simulink model "TV_2017"  (R2016a)
settings: Solver=FixedStepAuto  StartTime=0.0  StopTime=inf  FixedStep=0.001  RelTol=1e-3
PreLoadFcn:
  | TV_2017_parameters
values from neighbouring files (symbols this model uses):
  battery_voltage = single(530)    [HIL_parameters.m]    (also in HIL_parameters_2018.m; TV_2017_parameters.m; TV_2017_parameters_VD.m)
  car_params = Simulink_Car_params    [HIL_parameters.m]    (also in HIL_parameters_2018.m; TV_2017_parameters.m; TV_2017_parameters_VD.m)
  i_Diff = 16    [HIL_parameters.m]    (also in HIL_parameters_2018.m; TV_2017_parameters.m)
  Kp = 1    [HIL_parameters.m]    (also in HIL_parameters_2018.m; TV_2017_parameters.m; TV_2017_parameters_VD.m)
  motor_data = struct    [HIL_parameters.m]    (also in HIL_parameters_2018.m; TV_2017_parameters.m)
  powerLimitControl = Simulink_el    [HIL_parameters.m]    (also in HIL_parameters_2018.m; TV_2017_parameters.m; TV_2017_parameters_VD.m)
  settings = Simulink_Settings    [HIL_parameters.m]    (also in HIL_parameters_2018.m; TV_2017_parameters.m; TV_2017_parameters_VD.m)
  SpdC_BCC = 0    [HIL_parameters.m]    (also in HIL_parameters_2018.m; TV_2017_parameters.m; TV_2017_parameters_VD.m)
  Speed_Neg_sat = -21    [HIL_parameters.m]    (also in HIL_parameters_2018.m; TV_2017_parameters.m; TV_2017_parameters_VD.m)
  Speed_Pos_sat = 21    [HIL_parameters.m]    (also in HIL_parameters_2018.m; TV_2017_parameters.m; TV_2017_parameters_VD.m)
  SteeringAngleFL = [-23.80 -22.65 -21.50 -20.34 -19.18 -18.03 -16.86 -15.70 -14.53 -13.35 -12.18 -10.99 -9.80 -8.61 -7.40 -6.19 -4.97 -3.75 -2.51 -1.26 0 1.27 2.56 3.85 5.17 6.50 7.84 9.21 10.59 12.00 13.42 14.88 16.36 17.87 19.41 20.99 22.61 24.26 25.97 27.73 29.54]    [CarSetupAnalysis2018.m]    (also in HIL_parameters_2018.m; TV_2017_parameters.m; TV_2017_parameters_VD.m = [-24.129 -22.950 -21.772 -20.593 -19.413 -18.232 -17.050 -15)
  SteeringAngleFR = [-29.54 -27.73 -25.97 -24.26 -22.61 -20.99 -19.41 -17.87 -16.36 -14.88 -13.42 -12.00 -10.59 -9.21 -7.84 -6.50 -5.17 -3.85 -2.56 -1.27 0 1.26 2.51 3.75 4.97 6.19 7.40 8.61 9.80 10.99 12.18 13.35 14.53 15.70 16.86 18.03 19.18 20.34 21.50 22.65 23.80]    [CarSetupAnalysis2018.m]    (also in HIL_parameters_2018.m; TV_2017_parameters.m; TV_2017_parameters_VD.m = [-29.3050 -27.5340 -25.8140 -24.1410 -22.5110 -20.9180 -19.3)
  SteeringWhAngle = [-105 -99.75 -94.5 -89.25 -84 -78.75 -73.5 -68.25 -63 -57.75 -52.5 -47.25 -42 -36.75 -31.5 -26.25 -21.0 -15.75 -10.5 -5.25 0.0 5.25 10.50 15.75 21.00 26.25 31.50 36.75 42.00 47.25 52.50 57.75  63.00 68.25 73.50 78.75 84.00 89.25 94.50 99.75 105.00]    [TV_2017_parameters_VD.m]
  Tn_n = 0    [HIL_parameters.m]    (also in HIL_parameters_2018.m; TV_2017_parameters.m; TV_2017_parameters_VD.m)
  tractionControl = Simulink_tc    [HIL_parameters.m]    (also in HIL_parameters_2018.m; IterativeTractionControlTuning.m; TV_2017_parameters.m; TV_2017_parameters_VD.m)
  yawMomentGenerator = struct    [HIL_parameters.m]    (also in HIL_parameters_2018.m = Simulink_yawRate2; TV_2017_parameters.m = Simulink_yawRate2)
  yawRateControl = Simulink_yawRate    [HIL_parameters.m]    (also in HIL_parameters_2018.m; TV_2017_parameters.m; TV_2017_parameters_VD.m)
undefined symbols (not defined in the file or in its folder): DiscIntNeverNeededParam, magnitude, speedEstimation, TC_Decr_Gas, TC_Derivative, TC_Incr_Gas, TC_On, TC_Relay_Off, TC_Relay_On
libraries: CarMaker4SL x350, simulink_extras x63, simulink x37, dspfdesign x2
(part 1 of 14)
settings Model: Creator=fh  LastModifiedBy=95fre
settings DataIOCC: LimitDataPoints=on  SaveFormat=Array  SignalLoggingSaveFormat=ModelDataLogs  SignalLoggingName=sigsOut
settings OptimizationCC: DefaultUnderspecifiedDataType=single  OptimizeBlockIOStorage=off  BufferReuse=off  GlobalBufferReuse=off  ExpressionFolding=off  ExpressionDepthLimit=2147483647  LocalBlockOutputs=off  OptimizeModelRefInitCode=on  LifeSpan=Inf  MaxStackSize=64
settings DebuggingCC: SaveWithParameterizedLinksMsg=none  UnderspecifiedInitializationDetection=Classic  SignalResolutionControl=TryResolveAllWithWarning  MultiTaskDSMMsg=warning  MultiTaskCondExecSysMsg=none  BusObjectLabelMismatch=error  ModelReferenceVersionMismatchMessage=warning  StateNameClashWarn=warning
settings HardwareCC: ProdBitPerPointer=32  ProdLargestAtomicInteger=Long  ProdLargestAtomicFloat=Double  ProdWordSize=32  ProdHWDeviceType=ARM Compatible->ARM Cortex  TargetLargestAtomicInteger=Long  TargetLargestAtomicFloat=Double  TargetEndianess=LittleEndian  TargetHWDeviceType=ARM Compatible->ARM Cortex
settings ModelReferenceCC: PropagateSignalLabelsOutOfModel=off
settings RTWCC: SystemTargetFile=ert.tlc  GenCodeOnly=on  TemplateMakefile=ert_default_tmf  GenerateReport=on  Toolchain=GNU Tools for ARM Embedded Processors  BuildConfiguration=Debug  IncludeHyperlinkInReport=on  LaunchReport=on
settings CodeAppCC: ForceParamTrailComments=on  IgnoreCustomStorageClasses=off  SimulinkDataObjDesc=on  SFDataObjDesc=on  MATLABFcnDesc=on  InsertBlockDesc=on  MATLABSourceComments=on  EnableCustomComments=on  ReqsInCode=on
settings ERTTargetCC: GenerateSampleERTMain=on  IncludeMdlTerminateFcn=off  MatFileLogging=on  SupportNonFinite=off  SupportComplex=off  SupportVariableSizeSignals=on  ERTCustomFileTemplate=example_file_process.tlc  SuppressUnreachableDefaultCases=off
settings ConfigComp: CovHTMLOptions=-sRT=1 -sVT=0 -aTS=1 -bRG=1 -bTC=1 -hTR=0 -nFC=0 -nFD=1 -scm=1 -bcm=1 -xEv=0 -xEM=0  CovModelRefEnable=Off  PSAutoStubLUT=off

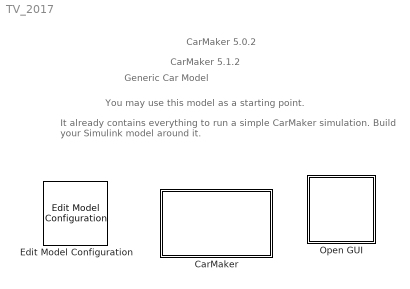
== system TV_2017 ==
  note: Generic Car Model
  note: You may use this model as a starting point.
  note: It already contains everything to run a simple CarMaker simulation.
      | Build your Simulink model around it.
  note: CarMaker 5.0.2
  note: CarMaker 5.1.2
  CarMaker : Subsystem  TreatAsAtomicUnit=on
      mask Display: image(imread('CarMakerSys.png'));
  Edit Model Configuration : CarMaker4SL/Edit Model Configuration
  Open GUI : Subsystem  LoadFcn=if ~length(which('cmcmd')), cmenv; end
      settings: OpenFcn=cmblockmagic('gui_fix_display'); CM_Simulink
      mask Display: image('CarMakerGUI.png');

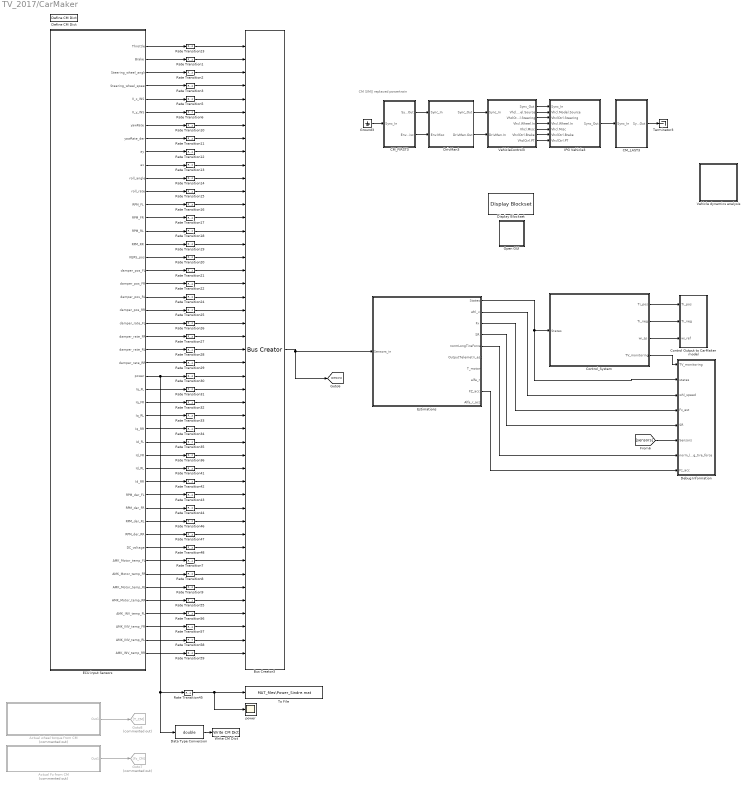
== system TV_2017/CarMaker ==
  note: CM SIM|| replaced powertrain
  Actual Fz from CM : Subsystem  Commented=on
  Actual wheel torque from CM : Subsystem  Commented=on
  Bus Creator3 : BusCreator  Inputs=47  OutDataTypeStr=Bus: SensorInputs  NonVirtualBus=on
      settings: InheritFromInputs=off
  CM_FIRST3 : Subsystem
  CM_LAST3 : Subsystem
  "Control Output to CarMaker model " : Subsystem
  "Control_System " : Subsystem  TreatAsAtomicUnit=on
  Data Type Conversion : DataTypeConversion  OutDataTypeStr=double
  "Debug Information " : Subsystem
  Define CM Dict : CarMaker4SL/Define CM Dict  xname=Power  xmono=off  xtype=Double  xdvaplace=None  xnstates=0  xfirststate=0  xinitial=0
  Display Blockset : CarMaker4SL/Display Blockset
  DrivMan3 : Subsystem
  "ECU input Sensors " : Subsystem  SystemSampleTime=settings.control_system_sample_time
  Estimations : Subsystem  TreatAsAtomicUnit=on
  Goto7 : Goto  Commented=on  GotoTag=Fz_CM
  Goto8 : Goto  Commented=on  GotoTag=T_CM
  Ground3 : Ground
  IPG Vehicle3 : Subsystem  TreatAsAtomicUnit=on
  Open GUI : Subsystem  LoadFcn=if ~length(which('cmcmd')), cmenv; end
      settings: OpenFcn=cmblockmagic('gui_fix_display'); CM_Simulink
      mask Display: image('CarMakerGUI.png');
  Rate Transition{1..3,5..36,41..48,55..59} (48 alike) : RateTransition  OutPortSampleTime=matlab_params.sensor_sampling_time
  Terminator3 : Terminator
  To File : ToFile  Filename=MAT_files\Power_Sindre.mat  MatrixName=Power  SaveFormat=Timeseries
  Vehicle dynamics analysis : Subsystem
  VehicleControl3 : Subsystem
  Write CM Dict : CarMaker4SL/Write CM Dict  xname=Power  xsync=off
  power : Scope
  wires:
  "Control_System "/1("Ti_pos ") -> "Control Output to CarMaker model "/1("Ti_pos ")
  "Control_System "/2(Ti_neg) -> "Control Output to CarMaker model "/2(Ti_neg)
  "Control_System "/3(wi_sp) -> "Control Output to CarMaker model "/3(wi_ref)
  Estimations/1(States) -> "Control_System "/1("States "), "Debug Information "/2(states)
  Estimations/2(whl_v) -> "Debug Information "/3(whl_speed)
  Estimations/3(Fx) -> "Debug Information "/4(Fx_est)
  Estimations/4(SR) -> "Debug Information "/5("SR ")
  Rate Transition45/1 -> power/1, To File/1
  "ECU input Sensors "/37(RPM_der_RL) -> Rate Transition46/1
  "ECU input Sensors "/38(RPM_der_RR) -> Rate Transition47/1
  "ECU input Sensors "/36(RPM_der_FR) -> Rate Transition44/1
  "ECU input Sensors "/35(RPM_der_FL) -> Rate Transition43/1
  "ECU input Sensors "/34(Id_RR) -> Rate Transition42/1
  "ECU input Sensors "/4(Steering_wheel_speed) -> Rate Transition3/1
  "ECU input Sensors "/1("Throttle ") -> Rate Transition23/1
  "ECU input Sensors "/2("Brake ") -> Rate Transition1/1
  "ECU input Sensors "/3("Steering_wheel_angle ") -> Rate Transition2/1
  "ECU input Sensors "/5(V_x_INS) -> Rate Transition5/1
  "ECU input Sensors "/6(V_y_INS) -> Rate Transition6/1
  "ECU input Sensors "/7(yawRate) -> Rate Transition10/1
  "ECU input Sensors "/9(ay) -> Rate Transition12/1
  "ECU input Sensors "/10("ax ") -> Rate Transition13/1
  "ECU input Sensors "/11(roll_angle) -> Rate Transition14/1
  "ECU input Sensors "/12(roll_rate) -> Rate Transition15/1
  "ECU input Sensors "/13(RPM_FL) -> Rate Transition16/1
  "ECU input Sensors "/14(RPM_FR) -> Rate Transition17/1
  "ECU input Sensors "/15(RPM_RL) -> Rate Transition18/1
  "ECU input Sensors "/16(RPM_RR) -> Rate Transition19/1
  "ECU input Sensors "/17(KERS_pos) -> Rate Transition20/1
  "ECU input Sensors "/18(damper_pos_FL) -> Rate Transition21/1
  "ECU input Sensors "/19(damper_pos_FR) -> Rate Transition22/1
  "ECU input Sensors "/20(damper_pos_RL) -> Rate Transition24/1
  "ECU input Sensors "/21(damper_pos_RR) -> Rate Transition25/1
  "ECU input Sensors "/22(damper_rate_FL) -> Rate Transition26/1
  "ECU input Sensors "/23(damper_rate_FR) -> Rate Transition27/1
  "ECU input Sensors "/24(damper_rate_RL) -> Rate Transition28/1
  "ECU input Sensors "/25(damper_rate_RR) -> Rate Transition29/1
  "ECU input Sensors "/27(Iq_FL) -> Rate Transition31/1
  "ECU input Sensors "/28(Iq_FR) -> Rate Transition32/1
  "ECU input Sensors "/29(Iq_RL) -> Rate Transition33/1
  "ECU input Sensors "/30(Iq_RR) -> Rate Transition34/1
  "ECU input Sensors "/31(Id_FL) -> Rate Transition35/1
  "ECU input Sensors "/32(Id_FR) -> Rate Transition36/1
  "ECU input Sensors "/33(Id_RL) -> Rate Transition41/1
  "ECU input Sensors "/8(yawRate_der) -> Rate Transition11/1
  "ECU input Sensors "/39(DC_voltage) -> Rate Transition48/1
  Rate Transition23/1 -> Bus Creator3/1
  Estimations/5(normLongTireForce) -> "Debug Information "/7(norm_long_tire_force)
  Rate Transition17/1 -> Bus Creator3/14
  Rate Transition12/1 -> Bus Creator3/9
  Rate Transition30/1 -> Bus Creator3/26
  Rate Transition14/1 -> Bus Creator3/11
  Rate Transition16/1 -> Bus Creator3/13
  Rate Transition25/1 -> Bus Creator3/21
  Rate Transition3/1 -> Bus Creator3/4
  Rate Transition2/1 -> Bus Creator3/3
  Rate Transition22/1 -> Bus Creator3/19
  Rate Transition11/1 -> Bus Creator3/8
  Rate Transition18/1 -> Bus Creator3/15
  Rate Transition20/1 -> Bus Creator3/17
  Rate Transition1/1 -> Bus Creator3/2
  Rate Transition24/1 -> Bus Creator3/20
  Rate Transition31/1 -> Bus Creator3/27
  Rate Transition26/1 -> Bus Creator3/22
  Rate Transition29/1 -> Bus Creator3/25
  Rate Transition15/1 -> Bus Creator3/12
  Rate Transition13/1 -> Bus Creator3/10
  Rate Transition28/1 -> Bus Creator3/24
  Rate Transition19/1 -> Bus Creator3/16
  Rate Transition21/1 -> Bus Creator3/18
  Rate Transition27/1 -> Bus Creator3/23
  Rate Transition6/1 -> Bus Creator3/6
  Rate Transition42/1 -> Bus Creator3/34
  Rate Transition47/1 -> Bus Creator3/38
  Rate Transition48/1 -> Bus Creator3/39
  Rate Transition41/1 -> Bus Creator3/33
  Rate Transition43/1 -> Bus Creator3/35
  Rate Transition35/1 -> Bus Creator3/31
  Rate Transition34/1 -> Bus Creator3/30
  Rate Transition46/1 -> Bus Creator3/37
  Rate Transition44/1 -> Bus Creator3/36
  Rate Transition33/1 -> Bus Creator3/29
  Rate Transition32/1 -> Bus Creator3/28
  Rate Transition36/1 -> Bus Creator3/32
  Rate Transition10/1 -> Bus Creator3/7
  Bus Creator3/1 -> [sensors], Estimations/1(Sensors_in)
  "ECU input Sensors "/26(power) -> Data Type Conversion/1, Rate Transition45/1, Rate Transition30/1
  Data Type Conversion/1 -> Write CM Dict/1
  [sensors] -> "Debug Information "/6(Sensors)
  "ECU input Sensors "/44(AMK_INV_temp_FL) -> Rate Transition56/1
  "ECU input Sensors "/40(AMK_Motor_temp_FL) -> Rate Transition7/1
  "ECU input Sensors "/41(AMK_Motor_temp_FR) -> Rate Transition8/1
  "ECU input Sensors "/42(AMK_Motor_temp_RL) -> Rate Transition9/1
  "ECU input Sensors "/43(AMK_Motor_temp_RR) -> Rate Transition55/1
  "ECU input Sensors "/45(AMK_INV_temp_FR) -> Rate Transition57/1
  "ECU input Sensors "/46(AMK_INV_temp_RL) -> Rate Transition58/1
  "ECU input Sensors "/47(AMK_INV_temp_RR) -> Rate Transition59/1
  Rate Transition7/1 -> Bus Creator3/40
  Rate Transition8/1 -> Bus Creator3/41
  Rate Transition9/1 -> Bus Creator3/42
  Rate Transition55/1 -> Bus Creator3/43
  Rate Transition56/1 -> Bus Creator3/44
  Rate Transition57/1 -> Bus Creator3/45
  Rate Transition58/1 -> Bus Creator3/46
  Rate Transition59/1 -> Bus Creator3/47
  Actual wheel torque from CM/1(Out1) -> Goto8/1
  Actual Fz from CM/1(Out1) -> Goto7/1
  "Control_System "/4(TV_monitoring) -> "Debug Information "/1(TV_monitoring)
  VehicleControl3/7(VhclCtrl.PT) -> IPG Vehicle3/7(VhclCtrl.PT)
  VehicleControl3/6(VhclCtrl.Brake) -> IPG Vehicle3/6(VhclCtrl.Brake)
  CM_FIRST3/1(Sync_Out) -> DrivMan3/1(Sync_In)
  CM_FIRST3/2(Env.Misc) -> DrivMan3/2(Env.Misc)
  VehicleControl3/3(VhclCtrl.Steering) -> IPG Vehicle3/3(VhclCtrl.Steering)
  DrivMan3/2(DrivMan.Out) -> VehicleControl3/2(DrivMan.In)
  VehicleControl3/2(Vhcl.Model.Source) -> IPG Vehicle3/2(Vhcl.Model.Source)
  VehicleControl3/5(Vhcl.Misc) -> IPG Vehicle3/5(Vhcl.Misc)
  VehicleControl3/1(Sync_Out) -> IPG Vehicle3/1(Sync_In)
  VehicleControl3/4(Vhcl.Wheel.In) -> IPG Vehicle3/4(Vhcl.Wheel.In)
  DrivMan3/1(Sync_Out) -> VehicleControl3/1(Sync_In)
  Ground3/1 -> CM_FIRST3/1(Sync_In)
  IPG Vehicle3/1(Sync_Out) -> CM_LAST3/1(Sync_In)
  CM_LAST3/1(Sync_Out) -> Terminator3/1
  Estimations/9(FZ_acc) -> "Debug Information "/8(Fz_acc)
  Rate Transition5/1 -> Bus Creator3/5

== system TV_2017/Open GUI ==
  S-Function : S-Function  FunctionName=cm_gui  SFunctionDeploymentMode=off  EnableBusSupport=off

== system TV_2017/CarMaker/Actual Fz from CM ==
  Bus Creator1 : BusCreator  Inputs=4
  Bus Creator4 : BusCreator  Inputs=4  OutDataTypeStr=Bus: normalForces  NonVirtualBus=on
      settings: InheritFromInputs=off
  Data Type Conversion{4..11} (8 alike) : DataTypeConversion  OutDataTypeStr=single
  Divide{,1..3} (4 alike) : Product  Inputs=*/
  Friction : Scope
  Rate Transition4 : RateTransition  OutPortSampleTime=matlab_params.sensor_sampling_time
  Read CM Dict10 : CarMaker4SL/Read CM Dict  xname=Vhcl.RL.Fx  xsync=off
  Read CM Dict11 : CarMaker4SL/Read CM Dict  xname=Vhcl.RR.Fx  xsync=off
  Read CM Dict3 : CarMaker4SL/Read CM Dict  xname=Vhcl.FR.Fz  xsync=off
  Read CM Dict4 : CarMaker4SL/Read CM Dict  xname=Vhcl.FL.Fz  xsync=off
  Read CM Dict5 : CarMaker4SL/Read CM Dict  xname=Vhcl.RR.Fz  xsync=off
  Read CM Dict6 : CarMaker4SL/Read CM Dict  xname=Vhcl.RL.Fz  xsync=off
  Read CM Dict8 : CarMaker4SL/Read CM Dict  xname=Vhcl.FL.Fx  xsync=off
  Read CM Dict9 : CarMaker4SL/Read CM Dict  xname=Vhcl.FR.Fx  xsync=off
  Out1 : Outport
  wires:
  Rate Transition4/1 -> Out1/1
  Read CM Dict4/1 -> Data Type Conversion4/1
  Read CM Dict5/1 -> Data Type Conversion7/1
  Read CM Dict3/1 -> Data Type Conversion5/1
  Read CM Dict6/1 -> Data Type Conversion6/1
  Data Type Conversion7/1 -> Bus Creator4/4, Divide3/2
  Data Type Conversion5/1 -> Bus Creator4/2, Divide1/2
  Data Type Conversion6/1 -> Bus Creator4/3, Divide2/2
  Divide/1 -> Bus Creator1/1  "FL"
  Read CM Dict10/1 -> Data Type Conversion10/1
  Data Type Conversion11/1 -> Divide3/1
  Data Type Conversion9/1 -> Divide1/1
  Data Type Conversion8/1 -> Divide/1
  Read CM Dict9/1 -> Data Type Conversion9/1
  Read CM Dict11/1 -> Data Type Conversion11/1
  Divide3/1 -> Bus Creator1/4  "RR"
  Bus Creator1/1 -> Friction/1
  Data Type Conversion4/1 -> Bus Creator4/1, Divide/2
  Read CM Dict8/1 -> Data Type Conversion8/1
  Divide2/1 -> Bus Creator1/3  "RL"
  Bus Creator4/1 -> Rate Transition4/1
  Data Type Conversion10/1 -> Divide2/1
  Divide1/1 -> Bus Creator1/2  "FR"

== system TV_2017/CarMaker/Actual wheel torque from CM ==
  Bus Creator2 : BusCreator  Inputs=4  OutDataTypeStr=Bus: T_meas
      settings: InheritFromInputs=off
  Data Type Conversion{1..3,12..15} (7 alike) : DataTypeConversion  OutDataTypeStr=single
  Rate Transition{37..40} (4 alike) : RateTransition  OutPortSampleTime=matlab_params.sensor_sampling_time
  Read CM Dict1 : CarMaker4SL/Read CM Dict  xname=Car.DampFL.Frc_tot  xsync=off
  Read CM Dict12 : CarMaker4SL/Read CM Dict  xname=PT.WFL.Trq_Drive  xsync=off
  Read CM Dict2 : CarMaker4SL/Read CM Dict  xname=Car.SpringFL.Frc_tot  xsync=off
  Read CM Dict45 : CarMaker4SL/Read CM Dict  xname=PT.WFR.Trq_Drive  xsync=off
  Read CM Dict46 : CarMaker4SL/Read CM Dict  xname=PT.WRL.Trq_Drive  xsync=off
  Read CM Dict47 : CarMaker4SL/Read CM Dict  xname=PT.WRR.Trq_Drive  xsync=off
  Read CM Dict7 : CarMaker4SL/Read CM Dict  xname=Car.StabiFL.Frc_tot  xsync=off
  "damp force fl " : Scope
  spring force fl : Scope
  spring force fl1 : Scope
  Out1 : Outport
  wires:
  Bus Creator2/1 -> Out1/1
  Rate Transition38/1 -> Bus Creator2/2
  Data Type Conversion1/1 -> "damp force fl "/1
  Data Type Conversion2/1 -> spring force fl/1
  Data Type Conversion3/1 -> spring force fl1/1
  Read CM Dict2/1 -> Data Type Conversion2/1
  Read CM Dict7/1 -> Data Type Conversion3/1
  Read CM Dict1/1 -> Data Type Conversion1/1
  Data Type Conversion12/1 -> Rate Transition37/1  "FL"
  Data Type Conversion14/1 -> Rate Transition39/1  "RL"
  Read CM Dict46/1 -> Data Type Conversion14/1
  Rate Transition39/1 -> Bus Creator2/3
  Data Type Conversion15/1 -> Rate Transition40/1  "RR"
  Read CM Dict12/1 -> Data Type Conversion12/1
  Read CM Dict47/1 -> Data Type Conversion15/1
  Rate Transition37/1 -> Bus Creator2/1
  Rate Transition40/1 -> Bus Creator2/4
  Read CM Dict45/1 -> Data Type Conversion13/1
  Data Type Conversion13/1 -> Rate Transition38/1  "FR"

== system TV_2017/CarMaker/CM_FIRST3 ==
  Sync_In : Inport
  BusCreator1 : BusCreator  Inputs=8
  BusCreator2 : BusCreator  Inputs=6
  Demux1 : Demux  Outputs=14
  Environment : S-Function  FunctionName=CM_Sfun  Parameters='Environment'  SFunctionDeploymentMode=off  EnableBusSupport=off
  IoIn : S-Function  FunctionName=CM_Sfun  Parameters='IoIn'  SFunctionDeploymentMode=off  EnableBusSupport=off
  Terminator : Terminator
  Sync_Out : Outport
  Env.Misc : Outport  Port=2
  wires:
  BusCreator2/1 -> Terminator/1  "IF Environment (in)"
  BusCreator1/1 -> Env.Misc/1
  Demux1/14 -> BusCreator2/6  "Env sRoad"
  Demux1/13 -> BusCreator2/5  "Env PoI_GCS Elev"
  Demux1/12 -> BusCreator2/4  "Env PoI_GCS Lat"
  Demux1/11 -> BusCreator2/3  "Env PoI_GCS Long"
  Demux1/10 -> BusCreator2/2  "Env Time"
  Demux1/9 -> BusCreator2/1  "Env yDay"
  Demux1/8 -> BusCreator1/8  "Env WindVel_tot z"
  Demux1/7 -> BusCreator1/7  "Env WindVel_tot y"
  Demux1/6 -> BusCreator1/6  "Env WindVel_tot x"
  Demux1/5 -> BusCreator1/5  "Env SolarRadiation"
  Demux1/4 -> BusCreator1/4  "Env AirHumidity"
  Demux1/3 -> BusCreator1/3  "Env AirPressure"
  Demux1/2 -> BusCreator1/2  "Env AirDensity"
  Demux1/1 -> BusCreator1/1  "Env Temperature"
  Environment/2 -> Demux1/1
  Environment/1 -> Sync_Out/1
  IoIn/1 -> Environment/1
  Sync_In/1 -> IoIn/1

== system TV_2017/CarMaker/CM_LAST3 ==
  Sync_In : Inport
  CM_User : S-Function  FunctionName=CM_Sfun  Parameters='CM_User'  SFunctionDeploymentMode=off  EnableBusSupport=off
  IoOut : S-Function  FunctionName=CM_Sfun  Parameters='IoOut'  SFunctionDeploymentMode=off  EnableBusSupport=off
  Sync_Out : Outport
  wires:
  IoOut/1 -> Sync_Out/1
  CM_User/1 -> IoOut/1
  Sync_In/1 -> CM_User/1

== system TV_2017/CarMaker/Control Output to CarMaker model  ==
  "Ti_pos " : Inport
  Ti_neg : Inport  Port=2
  wi_ref : Inport  Port=3
  Bus Selector : BusSelector  OutputSignals=FL,FR,RL,RR
  Bus Selector1 : BusSelector  OutputSignals=FL,FR,RL,RR
  Bus Selector2 : BusSelector  OutputSignals=FL,FR,RL,RR
  Data Type Conversion{,1..11} (12 alike) : DataTypeConversion  OutDataTypeStr=double
  Gain{,1..7} (8 alike) : Gain  Gain=car_params.Mn
  Scope4 : Scope
  Ti_To_CarMaker : Scope  NumInputPorts=4
  Write CM Dict : CarMaker4SL/Write CM Dict  xname=T_req_RR  xsync=off
  Write CM Dict1 : CarMaker4SL/Write CM Dict  xname=T_req_RL  xsync=off
  Write CM Dict10 : CarMaker4SL/Write CM Dict  xname=Tlim_pos_RL  xsync=off
  Write CM Dict11 : CarMaker4SL/Write CM Dict  xname=Tlim_pos_RR  xsync=off
  Write CM Dict16 : CarMaker4SL/Write CM Dict  xname=Tlim_neg_FL  xsync=off
  Write CM Dict17 : CarMaker4SL/Write CM Dict  xname=Tlim_neg_FR  xsync=off
  Write CM Dict18 : CarMaker4SL/Write CM Dict  xname=Tlim_neg_RL  xsync=off
  Write CM Dict19 : CarMaker4SL/Write CM Dict  xname=Tlim_neg_RR  xsync=off
  Write CM Dict2 : CarMaker4SL/Write CM Dict  xname=T_req_FR  xsync=off
  Write CM Dict3 : CarMaker4SL/Write CM Dict  xname=T_req_FL  xsync=off
  Write CM Dict4 : CarMaker4SL/Write CM Dict  xname=w_set_FR  xsync=off
  Write CM Dict5 : CarMaker4SL/Write CM Dict  xname=w_set_RL  xsync=off
  Write CM Dict6 : CarMaker4SL/Write CM Dict  xname=w_set_RR  xsync=off
  Write CM Dict7 : CarMaker4SL/Write CM Dict  xname=Tlim_pos_FL  xsync=off
  Write CM Dict8 : CarMaker4SL/Write CM Dict  xname=w_set_FL  xsync=off
  Write CM Dict9 : CarMaker4SL/Write CM Dict  xname=Tlim_pos_FR  xsync=off
  wires:
  "Ti_pos "/1 -> Bus Selector/1
  Bus Selector/1 -> Data Type Conversion/1  "<FL>"
  Bus Selector/2 -> Data Type Conversion1/1  "<FR>"
  Bus Selector/3 -> Data Type Conversion2/1  "<RL>"
  Bus Selector/4 -> Data Type Conversion3/1  "<RR>"
  Data Type Conversion3/1 -> Gain3/1
  Bus Selector1/1 -> Data Type Conversion4/1  "<FL>"
  Bus Selector1/2 -> Data Type Conversion5/1  "<FR>"
  Bus Selector1/3 -> Data Type Conversion6/1  "<RL>"
  Bus Selector1/4 -> Data Type Conversion7/1  "<RR>"
  wi_ref/1 -> Bus Selector1/1
  Data Type Conversion4/1 -> Write CM Dict8/1
  Data Type Conversion5/1 -> Write CM Dict4/1
  Data Type Conversion6/1 -> Write CM Dict5/1
  Data Type Conversion7/1 -> Scope4/1, Write CM Dict6/1
  Data Type Conversion1/1 -> Gain1/1
  Data Type Conversion/1 -> Gain/1
  Data Type Conversion2/1 -> Gain2/1
  Ti_neg/1 -> Bus Selector2/1
  Bus Selector2/1 -> Data Type Conversion8/1  "<FL>"
  Bus Selector2/2 -> Data Type Conversion9/1  "<FR>"
  Bus Selector2/3 -> Data Type Conversion10/1  "<RL>"
  Bus Selector2/4 -> Data Type Conversion11/1  "<RR>"
  Data Type Conversion8/1 -> Gain4/1
  Data Type Conversion9/1 -> Gain5/1
  Data Type Conversion10/1 -> Gain6/1
  Data Type Conversion11/1 -> Gain7/1
  Gain/1 -> Write CM Dict3/1, Ti_To_CarMaker/1, Write CM Dict7/1
  Gain1/1 -> Ti_To_CarMaker/2, Write CM Dict9/1, Write CM Dict2/1
  Gain2/1 -> Ti_To_CarMaker/3, Write CM Dict10/1, Write CM Dict1/1
  Gain3/1 -> Ti_To_CarMaker/4, Write CM Dict11/1, Write CM Dict/1
  Gain4/1 -> Write CM Dict16/1
  Gain5/1 -> Write CM Dict17/1
  Gain6/1 -> Write CM Dict18/1
  Gain7/1 -> Write CM Dict19/1

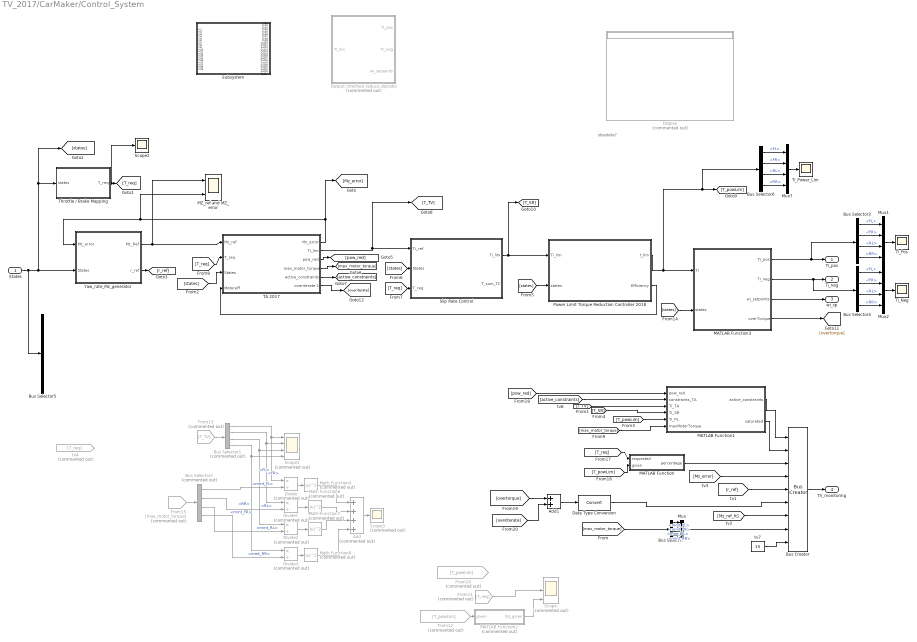
== system TV_2017/CarMaker/Control_System  ==
  note: obsolete?
  "States " : Inport
  Add : Sum  Commented=on  Inputs=++++
  Add1 : Sum
  Bus Creator : BusCreator  Inputs=9  OutDataTypeStr=Bus: TV_monitoring
      settings: InheritFromInputs=off
  Bus Selector : BusSelector  OutputSignals=mmt_FL,mmt_FR,mmt_RL,mmt_RR
  Bus Selector1 : BusSelector  Commented=on  OutputSignals=FL,FR,RL,RR
  Bus Selector2 : BusSelector  Commented=on  OutputSignals=mmt_FL,mmt_FR,mmt_RL,mmt_RR
  Bus Selector3 : BusSelector  OutputSignals=FL,FR,RL,RR
  Bus Selector4 : BusSelector  OutputSignals=FL,FR,RL,RR
  Bus Selector5 : BusSelector  OutputSignals=ax
  Bus Selector6 : BusSelector  OutputSignals=FL,FR,RL,RR
  Data Type Conversion : DataTypeConversion
  Display : Display  Commented=on
  Divide{,1..3} (4 alike) : Product  Commented=on  Inputs=*/
  From10 : From  Commented=on  GotoTag=T_powLim
  From11 : From  Commented=on  GotoTag=T_req
  From12 : From  Commented=on  GotoTag=T_powLim
  From13 : From  Commented=on  GotoTag=T_TV
  From15 : From  Commented=on  GotoTag=max_motor_torque
  MATLAB Function : MATLAB Function  TreatAsAtomicUnit=on
  MATLAB Function1 : MATLAB Function  TreatAsAtomicUnit=on
  MATLAB Function2 : MATLAB Function  Commented=on  TreatAsAtomicUnit=on
  MATLAB Function3 : MATLAB Function  TreatAsAtomicUnit=on
  MZ_ref and MZ_error : Scope  NumInputPorts=2
  Math Function{4,6..8} (4 alike) : Math  Commented=on  Operator=magnitude^2  SaturateOnIntegerOverflow=on
  Mux{,1..2,7} (4 alike) : Mux
  Output Interface reduce slipratio : Subsystem  Commented=on
  Power Limit Torque Reduction Controller 2018 : Subsystem
  Scope : Scope  Commented=on  NumInputPorts=3
  Scope1 : Scope  Commented=on  NumInputPorts=4
  Scope2 : Scope
  Scope3 : Scope  Commented=on
  "Slip Rate Control " : Subsystem
  Subsystem : Subsystem
  TA 2017 : Subsystem
  Throttle / Brake Mapping : MATLAB Function  TreatAsAtomicUnit=on
  Ti_Neg : Scope
  Ti_Pos : Scope
  Ti_Power_Lim : Scope
  Yaw_rate_Mz_generator : Subsystem
  tv4 : From  Commented=on  GotoTag=T_req
  tv7 : Constant  Value=15  OutDataTypeStr=single
  "Ti_pos " : Outport
  Ti_neg : Outport  Port=2
  wi_sp : Outport  Port=3
  TV_monitoring : Outport  Port=4
  wires:
  Throttle / Brake Mapping/1(T_req) -> Scope2/1, [T_req]
  TA 2017/1("Mz_error ") -> [Mz_error], MZ_ref and MZ_error/2, Yaw_rate_Mz_generator/1(Mz_error)
  [states] -> TA 2017/3("States ")
  TA 2017/2(Ti_lim) -> "Slip Rate Control "/1(Ti_ref), [T_TV]
  [states] -> Power Limit Torque Reduction Controller 2018/2(states)
  [T_req] -> TA 2017/2(T_req)
  "States "/1 -> Bus Selector5/1, [states], Throttle / Brake Mapping/1(states), Yaw_rate_Mz_generator/2(States)
  Bus Creator/1 -> TV_monitoring/1
  TA 2017/3(pow_red) -> [pow_red]
  [active_constraints] -> MATLAB Function1/2(constraints_TA)
  TA 2017/4(max_motor_torque) -> [max_motor_torque]
  TA 2017/5(active_constraints) -> [active_constraints]
  [pow_red] -> MATLAB Function1/1(pow_red)
  [T_powLim] -> MATLAB Function/2(given)
  [T_req] -> MATLAB Function/1(requested)
  [Mz_error] -> Bus Creator/4
  MATLAB Function/1(percentage) -> Bus Creator/3
  tv7/1 -> Bus Creator/9
  [max_motor_torque] -> Bus Selector/1
  [Mz_ref_tt] -> Bus Creator/7
  [r_ref] -> Bus Creator/5
  Add1/1 -> Data Type Conversion/1
  MATLAB Function3/3(wi_setpoints) -> wi_sp/1
  MATLAB Function3/1(Ti_pos) -> Bus Selector3/1, "Ti_pos "/1
  MATLAB Function3/2(Ti_neg) -> Bus Selector4/1, Ti_neg/1
  Mux/1 -> Bus Creator/8
  Bus Selector/1 -> Mux/1  "<mmt_FL>"
  Bus Selector/2 -> Mux/2  "<mmt_FR>"
  Bus Selector/3 -> Mux/3  "<mmt_RL>"
  Bus Selector/4 -> Mux/4  "<mmt_RR>"
  [states] -> "Slip Rate Control "/2("States ")
  [T_req] -> "Slip Rate Control "/3(T_req)
  "Slip Rate Control "/1(Ti_lim) -> [T_SR], Power Limit Torque Reduction Controller 2018/1(Ti_lim)
  [T_TV] -> MATLAB Function1/3(Ti_TA)
  [T_powLim] -> MATLAB Function1/5(Ti_PL)
  [T_SR] -> MATLAB Function1/4(Ti_SR)
  [max_motor_torque] -> MATLAB Function1/6(maxMotorTorque)
  MATLAB Function1/2(saturated) -> Bus Creator/2
  From11/1 -> Scope/2
  From12/1 -> MATLAB Function2/1(given)
  MATLAB Function2/1(tot_given) -> Scope/3
  From13/1 -> Bus Selector1/1
  Bus Selector1/1 -> Divide/1, Scope1/1  "<FL>"
  Bus Selector1/2 -> Divide1/1, Scope1/2  "<FR>"
  Bus Selector1/3 -> Divide2/1, Scope1/3  "<RL>"
  Bus Selector1/4 -> Divide3/1, Scope1/4  "<RR>"
  MATLAB Function1/1(active_constraints) -> Bus Creator/1
  Bus Selector2/1 -> Divide/2  "<mmt_FL>"
  Bus Selector2/2 -> Divide1/2  "<mmt_FR>"
  Bus Selector2/3 -> Divide2/2  "<mmt_RL>"
  Bus Selector2/4 -> Divide3/2  "<mmt_RR>"
  From15/1 -> Bus Selector2/1
  Divide/1 -> Math Function4/1
  Divide1/1 -> Math Function6/1
  Divide2/1 -> Math Function7/1
  Divide3/1 -> Math Function8/1
  Math Function4/1 -> Add/1
  Math Function6/1 -> Add/2
  Math Function7/1 -> Add/3
  Math Function8/1 -> Add/4
  Add/1 -> Scope3/1
  [states] -> MATLAB Function3/2(states)
  Power Limit Torque Reduction Controller 2018/1(t_lim) -> Bus Selector6/1, [T_powLim], MATLAB Function3/1(Ti)
  MATLAB Function3/4(overTorque) -> [overtorque]
  TA 2017/6(overiterate 1) -> [overiterate]
  [overtorque] -> Add1/1
  [overiterate] -> Add1/2
  Data Type Conversion/1 -> Bus Creator/6
  Bus Selector6/1 -> Mux7/1  "<FL>"
  Bus Selector6/2 -> Mux7/2  "<FR>"
  Bus Selector6/3 -> Mux7/3  "<RL>"
  Bus Selector6/4 -> Mux7/4  "<RR>"
  Mux7/1 -> Ti_Power_Lim/1
  Bus Selector3/1 -> Mux1/1  "<FL>"
  Bus Selector3/2 -> Mux1/2  "<FR>"
  Bus Selector3/3 -> Mux1/3  "<RL>"
  Bus Selector3/4 -> Mux1/4  "<RR>"
  Mux1/1 -> Ti_Pos/1
  Bus Selector4/1 -> Mux2/1  "<FL>"
  Bus Selector4/2 -> Mux2/2  "<FR>"
  Bus Selector4/3 -> Mux2/3  "<RL>"
  Bus Selector4/4 -> Mux2/4  "<RR>"
  Mux2/1 -> Ti_Neg/1
  Yaw_rate_Mz_generator/1(Mz_Ref) -> MZ_ref and MZ_error/1, TA 2017/1(Mz_ref)
  Yaw_rate_Mz_generator/2(r_ref) -> [r_ref]
  Power Limit Torque Reduction Controller 2018/2(Efficiency) -> TA 2017/4("Motoreff ")
